simulink model "Calc_wheel_speed"  (R2020b)
settings: Solver=ode45  StartTime=0.0  StopTime=25  MaxStep=0.01  RelTol=1e-3  AbsTol=1e-6
values from neighbouring files (symbols this model uses):
  I = 5.0    [abs_data_dict.sldd]
  Kf = 1.0    [abs_data_dict.sldd]
  PBmax = 1500.0    [abs_data_dict.sldd]
  Rr = 1.25    [abs_data_dict.sldd]
  TB = 0.01    [abs_data_dict.sldd]
  v0 = 88.0    [abs_data_dict.sldd]
settings Model: DataDictionary=abs_data_dict.sldd  Creator=nadee  LastModifiedBy=nadee
settings SolverCC: AutoScaleAbsTol=off
settings DataIOCC: SaveOutput=off  SaveTime=off

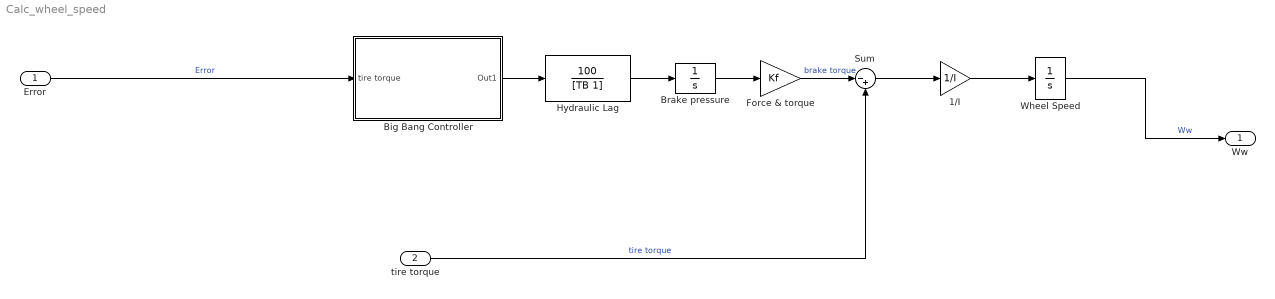
== system Calc_wheel_speed ==
  Error : Inport  OutDataTypeStr=double  PortDimensions=1  SampleTime=0
  tire torque : Inport  Port=2  OutDataTypeStr=double  PortDimensions=1  SampleTime=0
  1/I : Gain  Gain=1/I  SaturateOnIntegerOverflow=on  OutDataTypeStr=Inherit: Same as input  ParamDataTypeStr=Inherit: Same as input
  Big Bang Controller : Subsystem
  Brake pressure : Integrator  LimitOutput=on  UpperSaturationLimit=PBmax  LowerSaturationLimit=0
  Force & torque : Gain  Gain=Kf  SaturateOnIntegerOverflow=on  OutDataTypeStr=Inherit: Same as input  ParamDataTypeStr=Inherit: Same as input
  "Hydraulic Lag " : TransferFcn  Numerator=[100]  Denominator=[TB 1]
  Sum : Sum  Inputs=|-+  InputSameDT=on  SaturateOnIntegerOverflow=on  OutDataTypeStr=Inherit: Same as first input
  Wheel Speed : Integrator  InitialCondition=v0/Rr  LimitOutput=on  UpperSaturationLimit=1000  LowerSaturationLimit=0
  Ww : Outport  OutDataTypeStr=double  PortDimensions=1  SampleTime=0
  wires:
  Error/1 -> Big Bang Controller/1(tire torque)  "Error"
  1/I/1 -> Wheel Speed/1
  Sum/1 -> 1/I/1
  "Hydraulic Lag "/1 -> Brake pressure/1
  Wheel Speed/1 -> Ww/1  "Ww"
  tire torque/1 -> Sum/2  "tire torque"
  Force & torque/1 -> Sum/1  "brake torque"
  Big Bang Controller/1(Out1) -> "Hydraulic Lag "/1
  Brake pressure/1 -> Force & torque/1

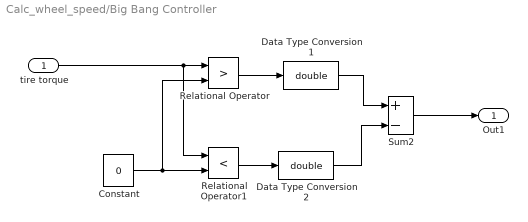
== system Calc_wheel_speed/Big Bang Controller ==
  tire torque : Inport
  Constant : Constant  Value=0
  Data Type Conversion1 : DataTypeConversion  OutDataTypeStr=double  SaturateOnIntegerOverflow=on  RndMeth=Zero
  Data Type Conversion2 : DataTypeConversion  OutDataTypeStr=double  SaturateOnIntegerOverflow=on  RndMeth=Zero
  Relational Operator : RelationalOperator  Operator=>  OutDataTypeStr=boolean  RndMeth=Nearest  InputSameDT=on
  Relational Operator1 : RelationalOperator  Operator=<  OutDataTypeStr=boolean  RndMeth=Nearest  InputSameDT=on
  Sum2 : Sum  Inputs=+-  InputSameDT=on  SaturateOnIntegerOverflow=on  OutDataTypeStr=Inherit: Same as first input
  Out1 : Outport
  wires:
  Sum2/1 -> Out1/1
  Relational Operator/1 -> Data Type Conversion1/1
  Data Type Conversion1/1 -> Sum2/1
  tire torque/1 -> Relational Operator/1, Relational Operator1/1
  Data Type Conversion2/1 -> Sum2/2
  Relational Operator1/1 -> Data Type Conversion2/1
  Constant/1 -> Relational Operator1/2, Relational Operator/2
